simulink model "exampleHeatTransfer2Ground"  (R2018b)
settings: Solver=ode45  StartTime=0.0  StopTime=365*24*3600  MaxStep=24*3600  RelTol=1e-3  EnableMultiTasking=on
libraries: carnot x1
settings Model: Creator=drhf  LastModifiedBy=drhf
settings DataIOCC: LimitDataPoints=on  SaveFormat=Array  SignalLoggingSaveFormat=ModelDataLogs
settings OptimizationCC: ExpressionDepthLimit=2147483647  LifeSpan=inf
settings DebuggingCC: UnderspecifiedInitializationDetection=Classic  MergeDetectMultiDrivingBlocksExec=none  SolverPrmCheckMsg=warning  StateNameClashWarn=warning  SFUnexpectedBacktrackingDiag=warning  SFNoUnconditionalDefaultTransitionDiag=warning  SFExecutionAtInitializationDiag=none
settings HardwareCC: ProdBitPerPointer=32  ProdBitPerSizeT=32  ProdBitPerPtrDiffT=32  ProdLargestAtomicFloat=None  ProdIntDivRoundTo=Undefined  ProdEndianess=Unspecified  ProdWordSize=32  ProdHWDeviceType=32-bit Generic
settings ModelReferenceCC: PropagateSignalLabelsOutOfModel=off
settings SFSimCC: SimUseLocalCustomCode=off
settings RTWCC: RTWUseLocalCustomCode=off
settings CodeAppCC: StateflowObjectComments=on
settings GRTTargetCC: TargetLangStandard=C89/C90 (ANSI)  GeneratePreprocessorConditionals=Disable all  CombineOutputUpdateFcns=off  GRTInterface=on
settings ConfigComp: CovMetricSettings=dw  CovHtmlReporting=on  CovSaveCumulativeToWorkspaceVar=on  CovSaveSingleToWorkspaceVar=on  CovExternalEMLEnable=off

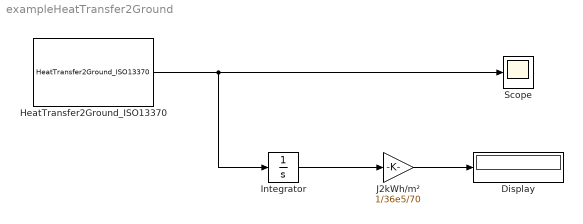
== system exampleHeatTransfer2Ground ==
  Display : Display
  HeatTransfer2Ground_ISO13370 : carnot/Basic/Heat_Transfer/HeatTransfer2Ground_ISO13370  slabwidth=10  slablength=7  gammat=0  Tmeaninside=23.8  deltathetai=3.8  Tmeanoutside=11  deltathetae=9.3  tshift=13.3*24*3600  dwall=0.4  cond_ground=2.0  cp_ground=800  rho_ground=2500  utot=0.183
  Integrator : Integrator
  J2kWh/m² : Gain  Gain=1/36e5/70
  Scope : Scope
  wires:
  HeatTransfer2Ground_ISO13370/1 -> Scope/1, Integrator/1
  Integrator/1 -> J2kWh/m²/1
  J2kWh/m²/1 -> Display/1
